simulink model "Regler_LQR"  (R2026a)
settings: Solver=ode23s  StartTime=tSim(1)  StopTime=tSim(end)  FixedStep=tStep  EnableMultiTasking=on
values from neighbouring files (symbols this model uses):
  Aobs = Fobs    [A4_4.m]
  Bobs = [E1 E2 Lobs]    [A4_4.m]
  Cobs = eye(4)    [A4_4.m]
  Dobs = zeros(4,3)    [A4_4.m]
  K = place(A, B, pK)    [A4_4.m]
  V = -1 / (Cx * ((A - B*K) \ B))    [A4_4.m]
  xhat0 = [0, 0, 0, 0]    [reglerInit.m]    (also in reglerInit_fin.m = [0; 0; 0; 0]; reglerInit_gain_scheduling.m; reglerInit_opt.m = [0; 0; 0; 0]; reglerInit_opt1.m = [0; 0; 0; 0])
undefined symbols (not defined in the file or in its folder): A_t, B_t, C_t, L_t, Mmax_total
settings Model: Creator=Henning Schlüter  LastModifiedBy=louis
settings DataIOCC: SignalLoggingSaveFormat=ModelDataLogs
settings DebuggingCC: UnderspecifiedInitializationDetection=Classic  PregeneratedLibrarySubsystemCodeDiagnostic=none
settings HardwareCC: ProdHWDeviceType=32-bit Generic
settings GRTTargetCC: CombineOutputUpdateFcns=off  GRTInterface=on

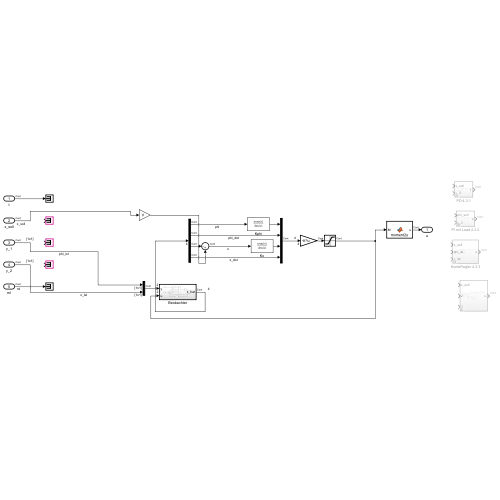
[thumbnail: Simulink's stored preview of the top-level diagram]
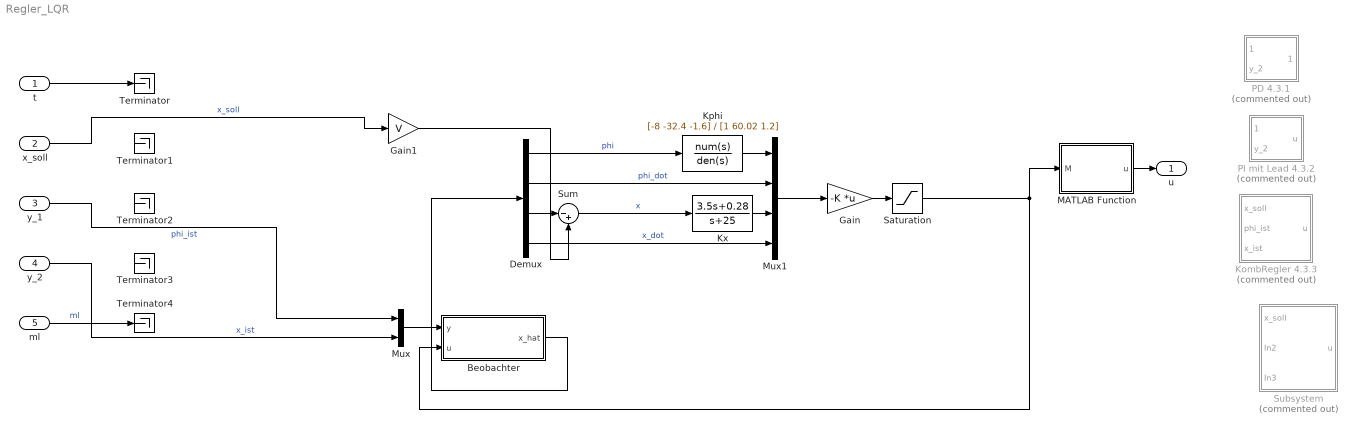
== system Regler_LQR ==
  t : Inport  OutDataTypeStr=double  PortDimensions=1  SampleTime=0
  "x_soll " : Inport  Port=2  OutDataTypeStr=double  PortDimensions=1  SampleTime=0
  y_1 : Inport  Port=3  OutDataTypeStr=double  PortDimensions=[1 1]  SampleTime=0
  y_2 : Inport  Port=4  OutDataTypeStr=double  PortDimensions=[1 1]  SampleTime=0
  ml : Inport  Port=5  OutDataTypeStr=double  PortDimensions=1  SampleTime=0
  Beobachter : Subsystem
  Demux : Demux
  Gain : Gain  Gain=-K  Multiplication=Matrix(K*u)
  Gain1 : Gain  Gain=V
  KombRegler 4.3.3 : Subsystem  Commented=on
  Kphi : TransferFcn  Numerator=[-8 -32.4 -1.6]  Denominator=[1 60.02 1.2]
  Kx : TransferFcn  Numerator=[3.5 0.28]  Denominator=[1 25]
  MATLAB Function : MATLAB Function  TreatAsAtomicUnit=on
  Mux : Mux  Inputs=2
  Mux1 : Mux
  PD 4.3.1 : Subsystem  Commented=on
  PI mit Lead 4.3.2 : Subsystem  Commented=on
  Saturation : Saturate  UpperLimit=Mmax_total  LowerLimit=-Mmax_total
  Subsystem : Subsystem  Commented=on
  Sum : Sum  Inputs=|-+
  Terminator{,1..4} (5 alike) : Terminator
  u : Outport  OutDataTypeStr=double  PortDimensions=1  VectorParamsAs1DForOutWhenUnconnected=off
  wires:
  t/1 -> Terminator/1
  ml/1 -> Terminator4/1  "ml"
  "x_soll "/1 -> Gain1/1  "x_soll"
  y_1/1 -> Mux/1  "phi_ist"
  y_2/1 -> Mux/2  "x_ist"
  Gain/1 -> Saturation/1
  Mux/1 -> Beobachter/1(y)
  Beobachter/1(x_hat) -> Demux/1
  Demux/3 -> Sum/1
  Sum/1 -> Kx/1  "x"
  Mux1/1 -> Gain/1
  Demux/4 -> Mux1/4  "x_dot"
  Demux/2 -> Mux1/2  "phi_dot"
  Demux/1 -> Kphi/1  "phi"
  Saturation/1 -> Beobachter/2(u), MATLAB Function/1(M)
  MATLAB Function/1(u) -> u/1
  Gain1/1 -> Sum/2
  Kphi/1 -> Mux1/1
  Kx/1 -> Mux1/3

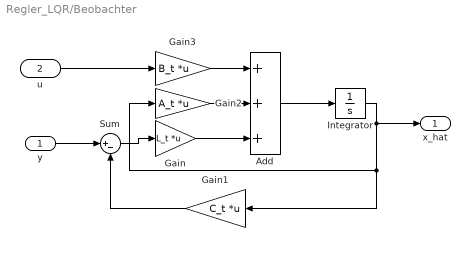
== system Regler_LQR/Beobachter ==
  y : Inport
  u : Inport  Port=2
  Add : Sum  Inputs=+++
  Gain : Gain  Gain=L_t  Multiplication=Matrix(K*u)
  Gain1 : Gain  Gain=C_t  Multiplication=Matrix(K*u)
  Gain2 : Gain  Gain=A_t  Multiplication=Matrix(K*u)
  Gain3 : Gain  Gain=B_t  Multiplication=Matrix(K*u)
  Integrator : Integrator  InitialCondition=xhat0
  Sum : Sum  Inputs=|+-
  x_hat : Outport
  wires:
  Add/1 -> Integrator/1
  Integrator/1 -> Gain2/1, Gain1/1, x_hat/1
  Sum/1 -> Gain/1
  Gain1/1 -> Sum/2
  y/1 -> Sum/1
  Gain/1 -> Add/3
  Gain2/1 -> Add/2
  Gain3/1 -> Add/1
  u/1 -> Gain3/1

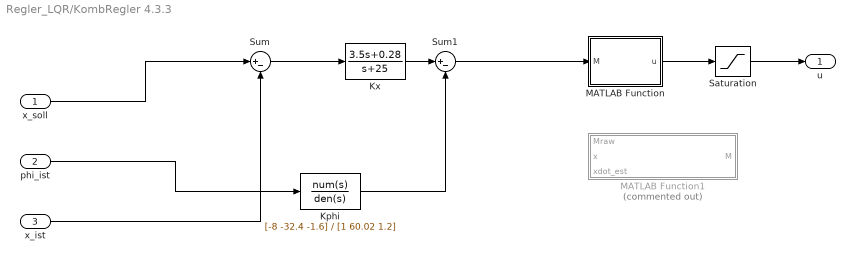
== system Regler_LQR/KombRegler 4.3.3 ==
  x_soll : Inport
  phi_ist : Inport  Port=2
  x_ist : Inport  Port=3
  Kphi : TransferFcn  Numerator=[-8 -32.4 -1.6]  Denominator=[1 60.02 1.2]
  Kx : TransferFcn  Numerator=[3.5 0.28]  Denominator=[1 25]
  MATLAB Function : MATLAB Function  TreatAsAtomicUnit=on
  MATLAB Function1 : MATLAB Function  Commented=on  TreatAsAtomicUnit=on
  Saturation : Saturate  UpperLimit=100  LowerLimit=-100
  Sum : Sum  Inputs=|+-
  Sum1 : Sum  Inputs=|+-
  u : Outport
  wires:
  MATLAB Function/1(u) -> Saturation/1
  x_soll/1 -> Sum/1
  Kphi/1 -> Sum1/2
  Sum1/1 -> MATLAB Function/1(M)
  Sum/1 -> Kx/1
  phi_ist/1 -> Kphi/1
  Kx/1 -> Sum1/1
  x_ist/1 -> Sum/2
  Saturation/1 -> u/1

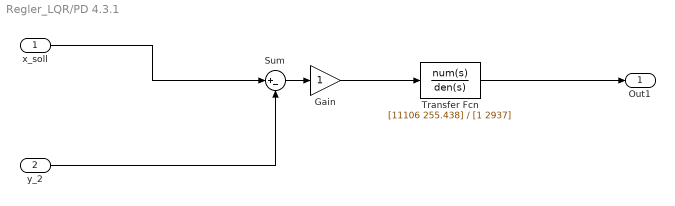
== system Regler_LQR/PD 4.3.1 ==
  x_soll : Inport
  y_2 : Inport  Port=2
  Gain : Gain
  Sum : Sum  Inputs=|+-
  Transfer Fcn : TransferFcn  Numerator=[11106 255.438]  Denominator=[1 2937]
  Out1 : Outport
  wires:
  Sum/1 -> Gain/1
  Gain/1 -> Transfer Fcn/1
  x_soll/1 -> Sum/1
  Transfer Fcn/1 -> Out1/1
  y_2/1 -> Sum/2

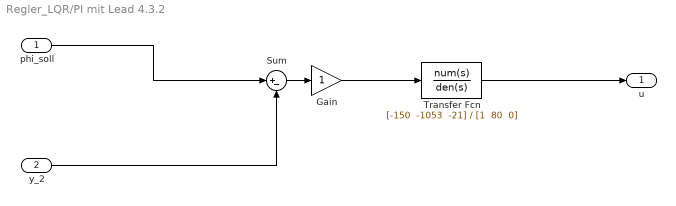
== system Regler_LQR/PI mit Lead 4.3.2 ==
  phi_soll : Inport
  y_2 : Inport  Port=2
  Gain : Gain
  Sum : Sum  Inputs=|+-
  Transfer Fcn : TransferFcn  Numerator="[-150  -1053  -21]"  Denominator="[1  80  0]"
  u : Outport
  wires:
  Sum/1 -> Gain/1
  Gain/1 -> Transfer Fcn/1
  phi_soll/1 -> Sum/1
  Transfer Fcn/1 -> u/1
  y_2/1 -> Sum/2

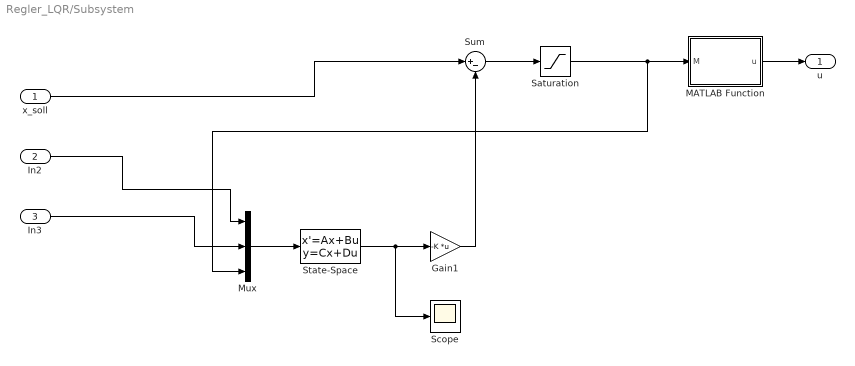
== system Regler_LQR/Subsystem ==
  x_soll : Inport
  In2 : Inport  Port=2
  In3 : Inport  Port=3
  Gain1 : Gain  Gain=-K  Multiplication=Matrix(K*u)
  MATLAB Function : MATLAB Function  TreatAsAtomicUnit=on
  Mux : Mux  Inputs=3
  Saturation : Saturate  UpperLimit=0.4  LowerLimit=-0.4
  Scope : Scope
      settings: ActiveDisplayYMinimum=-0.90880162510050011  ActiveDisplayYMaximum=0.44487709895687522
  State-Space : StateSpace  A=Aobs  B=Bobs  C=Cobs  D=Dobs  InitialCondition=[0, 0, 0, 0]
  Sum : Sum  Inputs=|+-
  u : Outport
  wires:
  MATLAB Function/1(u) -> u/1
  Sum/1 -> Saturation/1
  Saturation/1 -> Mux/3, MATLAB Function/1(M)
  In2/1 -> Mux/1
  Gain1/1 -> Sum/2
  Mux/1 -> State-Space/1
  State-Space/1 -> Scope/1, Gain1/1
  In3/1 -> Mux/2
  x_soll/1 -> Sum/1

== matlab function Regler_LQR/KombRegler 4.3.3/MATLAB Function ==
  data: M input; u output
function u = momentToU(M)
% Umrechnung Gesamtmoment M [Nm] in relative Motorleistung u [%]

% Zwei Motoren, je maximal 0.2 Nm
M = min(max(M, -0.4), 0.4);

% Inverse vereinfachte Motorkennlinie
u = 625 * sign(M) * M^2;

% Begrenzung auf Motorleistung
u = min(max(u, -100), 100);
end

== matlab function Regler_LQR/Subsystem/MATLAB Function ==
  data: M input; u output
function u = moment2u(M)
%#codegen

Pmax = 3.56;
Mmax_total = 0.4;

% Gesamtmoment begrenzen
M = min(max(M, -Mmax_total), Mmax_total);

% Gesamtmoment auf einen Motor
MM = M / 2;

% Inverse vereinfachte Motorkennlinie
P = sign(MM) * (9.434 * abs(MM))^2;

% Relative Leistung in Prozent
u = 100 * P / Pmax;

% Sicherheit
u = min(max(u, -100), 100);

end

== matlab function Regler_LQR/MATLAB Function ==
  data: M input; u output
function u = moment2u(M)
%#codegen

Pmax = 3.56;
Mmax_total = 0.4;

% Gesamtmoment begrenzen
M = min(max(M, -Mmax_total), Mmax_total);

% Gesamtmoment auf einen Motor
MM = M / 2;

% Inverse vereinfachte Motorkennlinie
P = sign(MM) * (9.434 * abs(MM))^2;

% Relative Leistung in Prozent
u = 100 * P / Pmax;

% Sicherheit
u = min(max(u, -100), 100);

end

== matlab function Regler_LQR/KombRegler 4.3.3/MATLAB Function1 ==
  data: Mraw input; M output; x input; xdot_est input
function M = safetyMoment(Mraw, x, xdot_est)
% Begrenzung und Wand-Sicherheit fuer das gewuenschte Gesamtmoment M [Nm]

% Grundbegrenzung
Mmax = 0.28;
M = min(max(Mraw, -Mmax), Mmax);

% Positionsgrenzen
xmin = -2.5;
xmax =  2.5;

% Sicherheitszone vor den Waenden
margin = 0.18;
xLowSoft  = xmin + margin;   % -2.32
xHighSoft = xmax - margin;   %  2.32

% Wandregler
Kwall = 1.2;
Dwall = 1.4;

% Untere Grenze:
% Wenn der Schlitten zu weit links ist, positives Moment erzwingen.
if x < xLowSoft
    Mwall = Kwall*(xLowSoft - x) - Dwall*xdot_est;
    M = max(M, Mwall);
end

% Obere Grenze:
% Wenn der Schlitten zu weit rechts ist, negatives Moment erzwingen.
if x > xHighSoft
    Mwall = Kwall*(xHighSoft - x) - Dwall*xdot_est;
    M = min(M, Mwall);
end

% Finale Begrenzung
M = min(max(M, -Mmax), Mmax);
end
